simulink model "course_hold_AP_2015"  (R2015a)
settings: Solver=ode45  SolverMode=SingleTasking  StartTime=0.0  StopTime=300  RelTol=1e-3
values from neighbouring files (symbols this model uses):
  alpha_fi1 = 2.87    [constants.m]    (also in prob_2_e.m)
  alpha_fi2 = -0.65    [constants.m]    (also in prob_2_e.m)
  g = 9.81    [constants.m]    (also in prob_2_e.m; rlocus.m = -h)
  kd_fi = (2*zeta_fi*omega_fi-alpha_fi1)/alpha_fi2    [constants.m]    (also in prob_2_e.m)
  ki_chi = omega_chi^2*V_g/g    [constants.m]    (also in prob_2_e.m)
  ki_fi = -0    (= 0)    [constants.m]    (also in prob_2_e.m)
  kp_chi = 2*zeta_chi*omega_chi*V_g/g    [constants.m]    (also in prob_2_e.m)
  kp_fi = -2    [constants.m]    (also in prob_2_e.m)
  V_g = 580/3.6    (= 161.111111111)    [constants.m]    (also in prob_2_e.m)
libraries: simulink_extras x2
settings Model: CovMetricSettings=dwe  CovHtmlReporting=off  covSaveCumulativeToWorkspaceVar=off  CovSaveSingleToWorkspaceVar=off  CovExternalEMLEnable=on  Creator=marti  LastModifiedBy=Anders Vagle
settings DataIOCC: LimitDataPoints=off  SaveFormat=Dataset
settings DebuggingCC: SFUnexpectedBacktrackingDiag=error  SFNoUnconditionalDefaultTransitionDiag=error
settings HardwareCC: ProdBitPerPointer=64  ProdLargestAtomicFloat=Float  ProdIntDivRoundTo=Zero  ProdEndianess=LittleEndian  ProdHWDeviceType=Specified
settings ModelReferenceCC: PropagateSignalLabelsOutOfModel=on
settings GRTTargetCC: TargetLangStandard=C99 (ISO)  GeneratePreprocessorConditionals=Use local settings

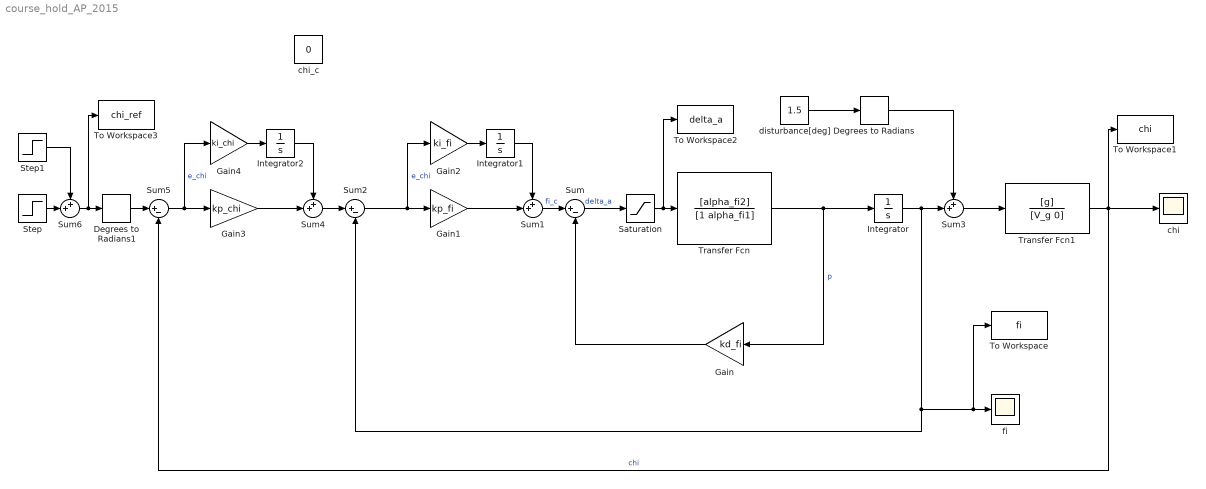
== system course_hold_AP_2015 ==
  Degrees to Radians : simulink_extras/Transformations/Degrees to Radians
  Degrees to Radians1 : simulink_extras/Transformations/Degrees to Radians
  Gain : Gain  Gain=kd_fi
  Gain1 : Gain  Gain=kp_fi
  Gain2 : Gain  Gain=ki_fi
  Gain3 : Gain  Gain=kp_chi
  Gain4 : Gain  Gain=ki_chi
  Integrator : Integrator
  Integrator1 : Integrator
  Integrator2 : Integrator
  Saturation : Saturate  UpperLimit=30/180*pi  LowerLimit=-30/180*pi
  Step : Step  Time=50  After=15  SampleTime=0
  Step1 : Step  Time=150  After=-15  SampleTime=0
  Sum : Sum  Inputs=|+-
  Sum{1,3..4,6} (4 alike) : Sum  Inputs=++|
  Sum2 : Sum  Inputs=|+-
  Sum5 : Sum  Inputs=|+-
  To Workspace : ToWorkspace  VariableName=fi  SaveFormat=Timeseries  SampleTime=-1
  To Workspace1 : ToWorkspace  VariableName=chi  SaveFormat=Timeseries  SampleTime=-1
  To Workspace2 : ToWorkspace  VariableName=delta_a  SaveFormat=Timeseries  SampleTime=-1
  To Workspace3 : ToWorkspace  VariableName=chi_ref  SaveFormat=Timeseries  SampleTime=-1
  Transfer Fcn : TransferFcn  Numerator=[alpha_fi2]  Denominator=[1 alpha_fi1]
  Transfer Fcn1 : TransferFcn  Numerator=[g]  Denominator=[V_g 0]
  chi : Scope
      settings: YMin=-10  YMax=10
  chi_c : Constant  Value=0
  disturbance[deg] : Constant  Value=1.5
  fi : Scope
      settings: YMin=-10  YMax=10
  wires:
  Transfer Fcn/1 -> Gain/1, Integrator/1  "p"
  Gain/1 -> Sum/2
  Gain2/1 -> Integrator1/1
  Sum1/1 -> Sum/1  "fi_c"
  Integrator1/1 -> Sum1/1
  Gain1/1 -> Sum1/2
  Sum2/1 -> Gain2/1, Gain1/1  "e_chi"
  Integrator/1 -> To Workspace/1, fi/1, Sum2/2, Sum3/2
  Sum3/1 -> Transfer Fcn1/1
  Transfer Fcn1/1 -> To Workspace1/1, Sum5/2, chi/1  "chi"
  Gain4/1 -> Integrator2/1
  Integrator2/1 -> Sum4/1
  Gain3/1 -> Sum4/2
  Sum5/1 -> Gain4/1, Gain3/1  "e_chi"
  Sum/1 -> Saturation/1  "delta_a"
  Saturation/1 -> To Workspace2/1, Transfer Fcn/1
  Sum4/1 -> Sum2/1
  Degrees to Radians1/1 -> Sum5/1
  disturbance[deg]/1 -> Degrees to Radians/1
  Degrees to Radians/1 -> Sum3/1
  Step/1 -> Sum6/2
  Sum6/1 -> To Workspace3/1, Degrees to Radians1/1
  Step1/1 -> Sum6/1
